simulink model "maglev"  (R2024a)
settings: Solver=VariableStepAuto  StartTime=0.0  StopTime=10.0  RelTol=1e-3
model mask{considerFem1=1, considerFem2=0, considerFd=0, considerFg=1, currentDynamicModel=1}
  mask prompts: considerFem1 "Upper inductance"; considerFem2 "Lower inductance"; considerFd "Aerodynamic drag"; considerFg "Gravity"
InitFcn:
  | run("plant\init.m")
model workspace (MAT data in the model file):
  considerFd = 0
  considerFem1 = 1
  considerFem2 = 0
  considerFg = 0
  currentDynamicModel = 1
values from neighbouring files (symbols this model uses):
  A = pi * r^2    (= 0.00294647029737)    [init.m]    (also in maglev_init.m)
  Cd = 0.45    [init.m]    (also in maglev_init.m)
  ci = 0.0243    [init.m]    (also in maglev_init.m)
  fiP1 = 1.4142 * 1e-4    (= 0.00014142)    [init.m]    (also in maglev_init.m)
  fiP2 = 4.5626 * 1e-3    (= 0.0045626)    [init.m]    (also in maglev_init.m)
  g = 9.81    [init.m]    (also in maglev_init.m)
  H = (75 + 61.25) * 1e-3    (= 0.13625)    [init.m]    (also in maglev_init.m = 0.098)
  ki = 2.5165    [init.m]    (also in maglev_init.m)
  m = 57.57 * 1e-3    (= 0.05757)    [init.m]
  rho = 1.21    [init.m]    (also in maglev_init.m)
undefined symbols (not defined in the file or in its folder): R10, R20, v0, z0
settings Model: ParameterArgumentNames=considerFd,considerFem1,considerFem2,considerFg,currentDynamicModel  Creator=Bocchio  LastModifiedBy=Bocchio

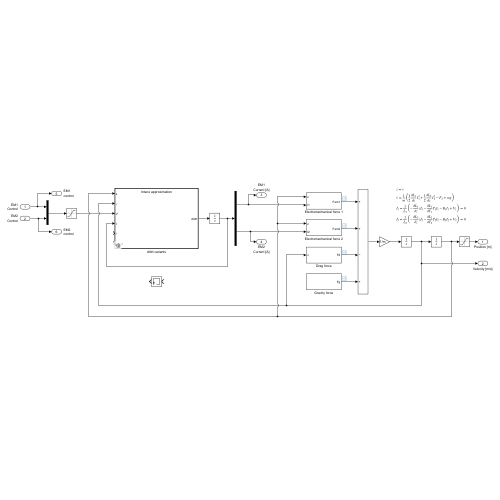
[thumbnail: Simulink's stored preview of the top-level diagram]
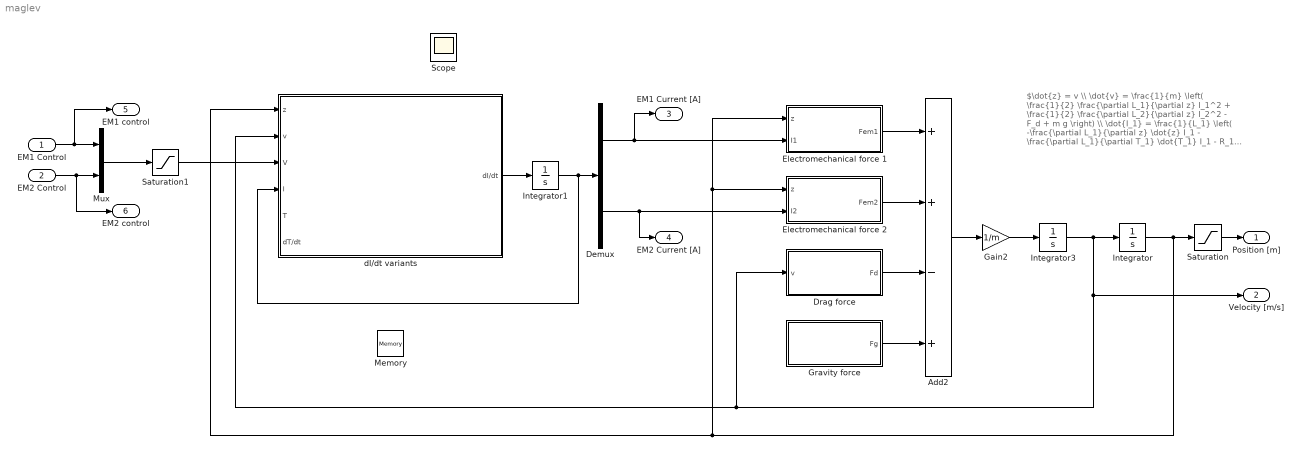
== system maglev ==
  note: $\dot{z} = v \\ \dot{v} = \frac{1}{m} \left( \frac{1}{2} \frac{\partial L_1}{\partial z} I_1^2 + \frac{1}{2} \frac{\partial L_2}{\partial z} I_2^2 - F_d + m g \right) \\ \dot{I_1} = \frac{1}{L_1} \left( -\frac{\partial L_1}{\partial z} \dot{z} I_1 - \frac{\partial L_1}{\partial T_1} \dot{T_1} I_1 - R_1 I_1 + V_1 \right) = 0 \\ \dot{I_2} = \frac{1}{L_2} \left( -\frac{\partial L_2}{\partial z} \dot{z} I_2 - \frac{\partial L_2}{\partial T_2} \dot{T_2} I_2 - R_2 I_2 + V_2 \right) = 0$
  EM1 Control : Inport
  EM2 Control : Inport  Port=2
  Add2 : Sum  Inputs=++-+
  Demux : Demux  Outputs=2
  Drag force : Subsystem
  Electromechanical force 1 : Subsystem
  Electromechanical force 2 : Subsystem
  Gain2 : Gain  Gain=1/m
  Gravity force : Subsystem
  Integrator : Integrator  InitialCondition=z0
  Integrator1 : Integrator  InitialCondition=ci
  Integrator3 : Integrator  InitialCondition=v0
  Memory : Memory  InitialCondition=ci
  Mux : Mux  Inputs=2
  Saturation : Saturate  UpperLimit=H  LowerLimit=0
  Saturation1 : Saturate  UpperLimit=1  LowerLimit=0
  dI/dt variants : Subsystem  Variant=on  VariantActivationTime=startup
  Position [m] : Outport
  Velocity [m/s] : Outport  Port=2
  EM1 Current [A] : Outport  Port=3
  EM2 Current [A] : Outport  Port=4
  EM1 control : Outport  Port=5
  EM2 control : Outport  Port=6
  Scope : Scope
  wires:
  Integrator/1 -> Saturation/1, dI/dt variants/1(z), Electromechanical force 1/1(z), Electromechanical force 2/1(z)
  Add2/1 -> Gain2/1
  Integrator3/1 -> Drag force/1(v), dI/dt variants/2(v), Velocity [m/s]/1, Integrator/1
  EM1 Control/1 -> EM1 control/1, Mux/1
  Gain2/1 -> Integrator3/1
  Demux/1 -> EM1 Current [A]/1, Electromechanical force 1/2(I1)
  Demux/2 -> EM2 Current [A]/1, Electromechanical force 2/2(I2)
  EM2 Control/1 -> EM2 control/1, Mux/2
  dI/dt variants/1(dI/dt) -> Integrator1/1
  Gravity force/1(Fg) -> Add2/4
  Drag force/1(Fd) -> Add2/3
  Electromechanical force 2/1(Fem2) -> Add2/2
  Electromechanical force 1/1(Fem1) -> Add2/1
  Saturation/1 -> Position [m]/1
  Mux/1 -> Saturation1/1
  Saturation1/1 -> dI/dt variants/3(V)
  Integrator1/1 -> dI/dt variants/4(I), Demux/1

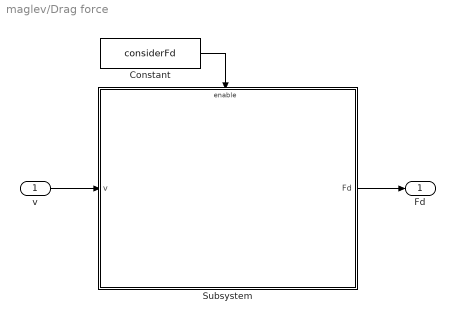
== system maglev/Drag force ==
  v : Inport
  Constant : Constant  Value=considerFd
  Subsystem : Subsystem
  Fd : Outport
  wires:
  v/1 -> Subsystem/1(v)
  Subsystem/1(Fd) -> Fd/1
  Constant/1 -> Subsystem/Enable

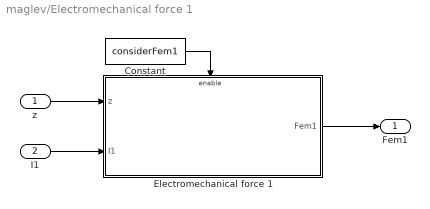
== system maglev/Electromechanical force 1 ==
  z : Inport
  I1 : Inport  Port=2
  Constant : Constant  Value=considerFem1
  Electromechanical force 1 : Subsystem  TreatAsAtomicUnit=on
  Fem1 : Outport
  wires:
  z/1 -> Electromechanical force 1/1(z)
  Electromechanical force 1/1(Fem1) -> Fem1/1
  Constant/1 -> Electromechanical force 1/Enable
  I1/1 -> Electromechanical force 1/2(I1)

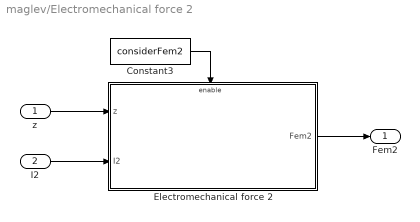
== system maglev/Electromechanical force 2 ==
  z : Inport
  I2 : Inport  Port=2
  Constant3 : Constant  Value=considerFem2
  Electromechanical force 2 : Subsystem  TreatAsAtomicUnit=on
  Fem2 : Outport
  wires:
  Constant3/1 -> Electromechanical force 2/Enable
  Electromechanical force 2/1(Fem2) -> Fem2/1
  z/1 -> Electromechanical force 2/1(z)
  I2/1 -> Electromechanical force 2/2(I2)

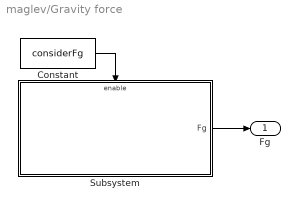
== system maglev/Gravity force ==
  Constant : Constant  Value=considerFg
  Subsystem : Subsystem
  Fg : Outport
  wires:
  Subsystem/1(Fg) -> Fg/1
  Constant/1 -> Subsystem/Enable

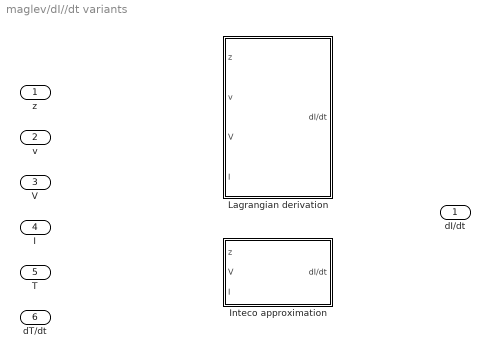
== system maglev/dI//dt variants ==
  z : Inport
  v : Inport  Port=2
  V : Inport  Port=3
  I : Inport  Port=4
  T : Inport  Port=5
  dT/dt : Inport  Port=6
  Inteco approximation : Subsystem  TreatAsAtomicUnit=on  VariantControl=currentDynamicModel==1
  Lagrangian derivation : Subsystem  TreatAsAtomicUnit=on  VariantControl=currentDynamicModel==2
  dI/dt : Outport

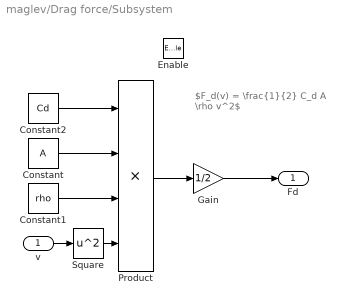
== system maglev/Drag force/Subsystem ==
  note: $F_d(v) = \frac{1}{2} C_d A \rho v^2$
  v : Inport
  Enable : EnablePort
  Constant : Constant  Value=A
  Constant1 : Constant  Value=rho
  Constant2 : Constant  Value=Cd
  Gain : Gain  Gain=1/2
  Product : Product  Inputs=4
  Square : Math  Operator=square
  Fd : Outport
  wires:
  v/1 -> Square/1
  Constant/1 -> Product/2
  Constant1/1 -> Product/3
  Constant2/1 -> Product/1
  Gain/1 -> Fd/1
  Product/1 -> Gain/1
  Square/1 -> Product/4

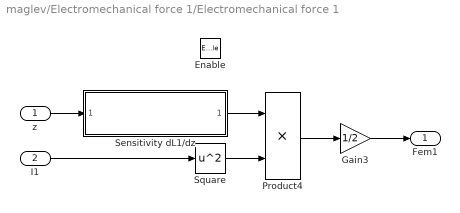
== system maglev/Electromechanical force 1/Electromechanical force 1 ==
  z : Inport
  I1 : Inport  Port=2
  Enable : EnablePort
  Gain3 : Gain  Gain=1/2
  Product4 : Product
  Sensitivity dL1/dz : Subsystem  ReferencedSubsystem=dL1dz
  Square : Math  Operator=square
  Fem1 : Outport
  wires:
  I1/1 -> Square/1
  Sensitivity dL1/dz/1 -> Product4/1
  Gain3/1 -> Fem1/1
  z/1 -> Sensitivity dL1/dz/1
  Product4/1 -> Gain3/1
  Square/1 -> Product4/2

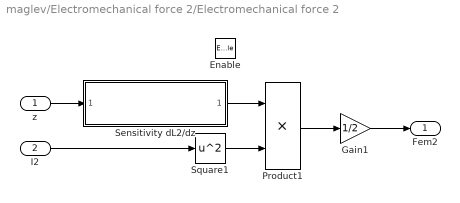
== system maglev/Electromechanical force 2/Electromechanical force 2 ==
  z : Inport
  I2 : Inport  Port=2
  Enable : EnablePort
  Gain1 : Gain  Gain=1/2
  Product1 : Product
  Sensitivity dL2/dz : Subsystem  ReferencedSubsystem=dL2dz
  Square1 : Math  Operator=square
  Fem2 : Outport  OutputWhenDisabled=reset  InitialOutput=0
  wires:
  Gain1/1 -> Fem2/1
  Sensitivity dL2/dz/1 -> Product1/1
  I2/1 -> Square1/1
  z/1 -> Sensitivity dL2/dz/1
  Product1/1 -> Gain1/1
  Square1/1 -> Product1/2

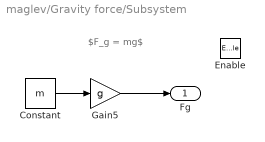
== system maglev/Gravity force/Subsystem ==
  note: $F_g = mg$
  Enable : EnablePort
  Constant : Constant  Value=m
  Gain5 : Gain  Gain=g
  Fg : Outport
  wires:
  Gain5/1 -> Fg/1
  Constant/1 -> Gain5/1

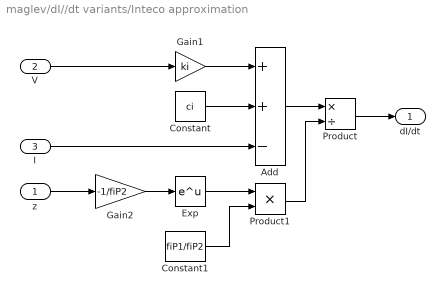
== system maglev/dI//dt variants/Inteco approximation ==
  z : Inport
  V : Inport  Port=2
  I : Inport  Port=3
  Add : Sum  Inputs=++-
  Constant : Constant  Value=ci
  Constant1 : Constant  Value=fiP1/fiP2
  Exp : Math
  Gain1 : Gain  Gain=ki
  Gain2 : Gain  Gain=-1/fiP2
  Product : Product  Inputs=*/
  Product1 : Product
  dI/dt : Outport
  wires:
  z/1 -> Gain2/1
  Exp/1 -> Product1/1
  I/1 -> Add/3
  Gain2/1 -> Exp/1
  V/1 -> Gain1/1
  Constant1/1 -> Product1/2
  Constant/1 -> Add/2
  Gain1/1 -> Add/1
  Add/1 -> Product/1
  Product1/1 -> Product/2
  Product/1 -> dI/dt/1

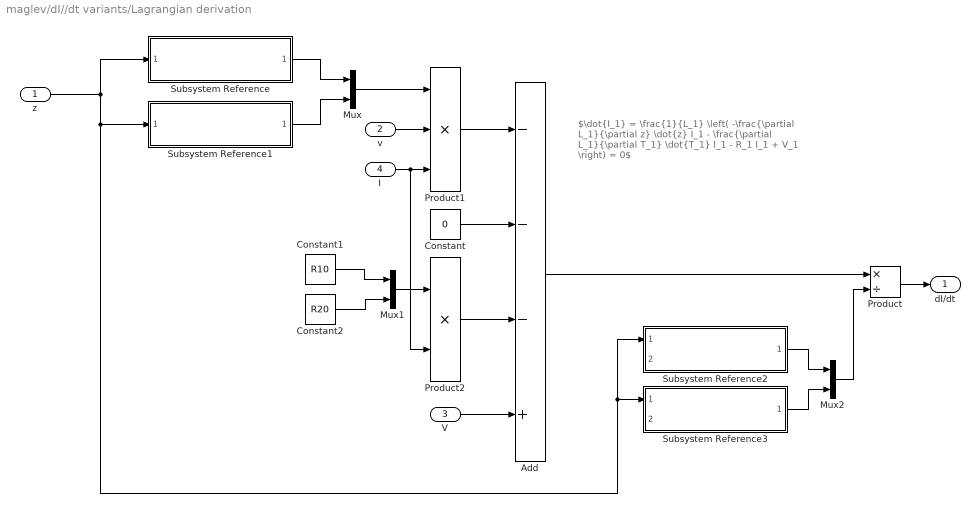
== system maglev/dI//dt variants/Lagrangian derivation ==
  note: $\dot{I_1} = \frac{1}{L_1} \left( -\frac{\partial L_1}{\partial z} \dot{z} I_1 - \frac{\partial L_1}{\partial T_1} \dot{T_1} I_1 - R_1 I_1 + V_1 \right) = 0$
  z : Inport
  v : Inport  Port=2
  V : Inport  Port=3
  I : Inport  Port=4
  Add : Sum  Inputs=---+
  Constant : Constant  Value=0
  Constant1 : Constant  Value=R10
  Constant2 : Constant  Value=R20
  Mux : Mux  Inputs=2
  Mux1 : Mux  Inputs=2
  Mux2 : Mux  Inputs=2
  Product : Product  Inputs=*/
  Product1 : Product  Inputs=3
  Product2 : Product
  Subsystem Reference : Subsystem  ReferencedSubsystem=dL1dz
  Subsystem Reference1 : Subsystem  ReferencedSubsystem=dL2dz
  Subsystem Reference2 : Subsystem  ReferencedSubsystem=L1
  Subsystem Reference3 : Subsystem  ReferencedSubsystem=L2
  dI/dt : Outport
  wires:
  Add/1 -> Product/1
  Product/1 -> dI/dt/1
  Mux2/1 -> Product/2
  z/1 -> Subsystem Reference2/1, Subsystem Reference3/1, Subsystem Reference1/1, Subsystem Reference/1
  Subsystem Reference/1 -> Mux/1
  Subsystem Reference1/1 -> Mux/2
  Mux/1 -> Product1/1
  v/1 -> Product1/2
  I/1 -> Product2/2, Product1/3
  Product1/1 -> Add/1
  Constant/1 -> Add/2
  Constant1/1 -> Mux1/1
  Constant2/1 -> Mux1/2
  Mux1/1 -> Product2/1
  Product2/1 -> Add/3
  V/1 -> Add/4
  Subsystem Reference2/1 -> Mux2/1
  Subsystem Reference3/1 -> Mux2/2
